simulink model "dyn_block"  (R2023b)
settings: Solver=VariableStepAuto  StartTime=0.0  StopTime=10.0  RelTol=1e-3
values from neighbouring files (symbols this model uses):
  i1 = sat.diaginertiamatrix(1, 1)    [set_params.m]
  i2 = sat.diaginertiamatrix(2, 2)    [set_params.m]
  i3 = sat.diaginertiamatrix(3, 3)    [set_params.m]
undefined symbols (not defined in the file or in its folder): compact, sat
libraries: aerolibutil x9, sharedtransform x2, shared6dof x1, sharedutil x1
settings Model: Creator=aryam  LastModifiedBy=aryam

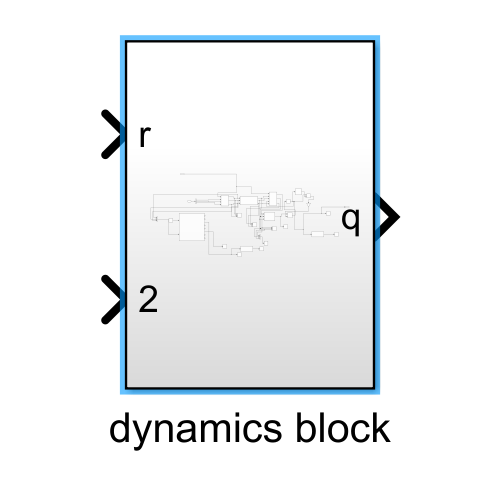
[thumbnail: Simulink's stored preview of the top-level diagram]
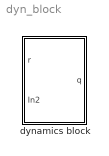
== system dyn_block ==
  dynamics block : Subsystem

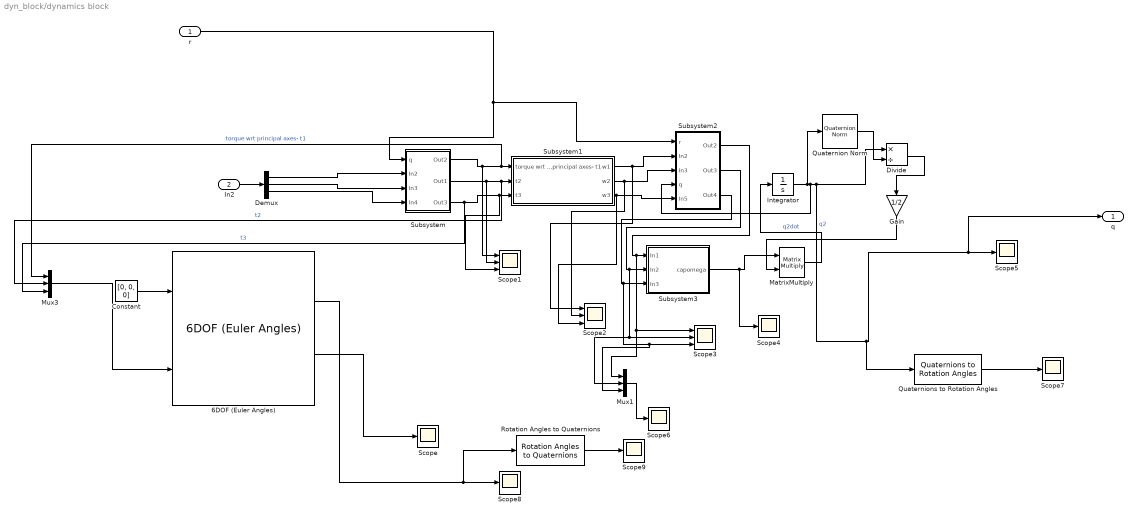
== system dyn_block/dynamics block ==
  r : Inport
  In2 : Inport  Port=2
  6DOF (Euler Angles) : shared6dof/6DOF (Euler Angles)  units=Metric (MKS)  mtype=Fixed  rep=Quaternion  xme_0=[0 0 0]  Vm_0=[0 0 0]  eul_0=[0 0 0]  pm_0=[0 0 0]  mass_0=1.0  mass_e=0.5  mass_f=2.0  inertia=sat.inertiamatrix  inertia_e=eye(3)  inertia_f=2*eye(3)  k_quat=1.0  vre_flag=on  abi_flag=off  aMode=0  xme_statename=''  Vm_statename=''  eul_statename=''  quat_statename=''  pm_statename=''  mass_statename=''
  Constant : Constant  Value=[0, 0, 0]
  Demux : Demux  Outputs=3
  Divide : Product  Inputs=*/
  Gain : Gain  Gain=1/2
  Integrator : Integrator  InitialCondition=compact(sat.initialorientation)
  MatrixMultiply : Product  Multiplication=Matrix(*)
  Mux1 : Mux  Inputs=3
  Mux3 : Mux  Inputs=3
  Quaternion Norm : sharedutil/Quaternion Norm  aMode=aMode
      settings: LibrarySourceBlock=|
      | aerolibutil/Quaternion
      | Norm
  Quaternions to Rotation Angles : sharedtransform/Quaternions to Rotation Angles  rotationOrder=ZYX  aMode=aMode
  Rotation Angles to Quaternions : sharedtransform/Rotation Angles to Quaternions  rotationOrder=ZYX  aMode=aMode
  Scope{,4..9} (7 alike) : Scope
  Scope1 : Scope  NumInputPorts=3
  Scope2 : Scope  NumInputPorts=3
  Scope3 : Scope  NumInputPorts=3
  Subsystem : Subsystem
  Subsystem1 : Subsystem
  Subsystem2 : Subsystem
  Subsystem3 : Subsystem
  q : Outport
  wires:
  Subsystem2/2(Out3) -> Scope3/2, Mux1/2, Subsystem3/2(In2)
  Subsystem2/3(Out4) -> Mux1/3, Scope3/3, Subsystem3/3(In3)
  Gain/1 -> MatrixMultiply/2
  Subsystem/1(Out2) -> Mux3/1, Subsystem1/1(torque wrt principal axes- t1), Scope1/1  "torque wrt principal axes- t1"
  Subsystem1/1(w1) -> Scope2/1, Subsystem2/2(In2)
  Subsystem3/1(capomega) -> Scope4/1, MatrixMultiply/1
  MatrixMultiply/1 -> Integrator/1  "q2dot"
  Subsystem/3(Out3) -> Mux3/3, Scope1/3, Subsystem1/3(t3)  "t3"
  r/1 -> Subsystem2/1(r), Subsystem/1(q)
  Subsystem1/2(w2) -> Scope2/2, Subsystem2/3(In3)
  Subsystem1/3(w3) -> Subsystem2/5(In5), Scope2/3
  Quaternion Norm/1 -> Divide/2
  Subsystem/2(Out1) -> Mux3/2, Subsystem1/2(t2), Scope1/2  "t2"
  Divide/1 -> Gain/1
  Integrator/1 -> Quaternions to Rotation Angles/1, q/1, Scope5/1, Divide/1, Subsystem2/4(q), Quaternion Norm/1  "q2"
  Subsystem2/1(Out2) -> Mux1/1, Scope3/1, Subsystem3/1(In1)
  Mux1/1 -> Scope6/1
  Mux3/1 -> 6DOF (Euler Angles)/2
  Constant/1 -> 6DOF (Euler Angles)/1
  6DOF (Euler Angles)/6 -> Scope/1
  Quaternions to Rotation Angles/1 -> Scope7/1
  6DOF (Euler Angles)/3 -> Rotation Angles to Quaternions/1, Scope8/1
  In2/1 -> Demux/1
  Demux/1 -> Subsystem/2(In2)
  Demux/2 -> Subsystem/3(In3)
  Demux/3 -> Subsystem/4(In4)
  Rotation Angles to Quaternions/1 -> Scope9/1

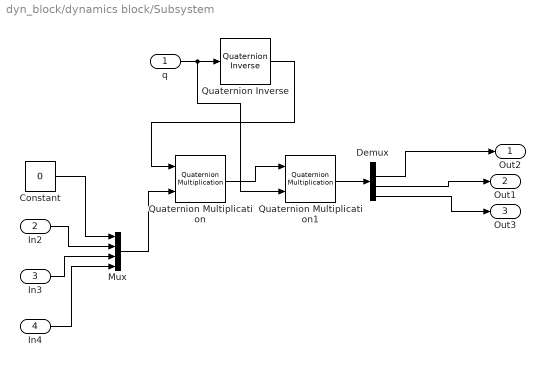
== system dyn_block/dynamics block/Subsystem ==
  q : Inport
  In2 : Inport  Port=2
  In3 : Inport  Port=3
  In4 : Inport  Port=4
  Constant : Constant  Value=0
  Demux : Demux
  Mux : Mux
  Quaternion Inverse : aerolibutil/Quaternion Inverse
  Quaternion Multiplication : aerolibutil/Quaternion Multiplication
  Quaternion Multiplication1 : aerolibutil/Quaternion Multiplication
  Out2 : Outport
  Out1 : Outport  Port=2
  Out3 : Outport  Port=3
  wires:
  Quaternion Multiplication/1 -> Quaternion Multiplication1/1
  Constant/1 -> Mux/1
  Mux/1 -> Quaternion Multiplication/2
  Demux/4 -> Out3/1
  q/1 -> Quaternion Multiplication1/2, Quaternion Inverse/1
  Quaternion Multiplication1/1 -> Demux/1
  Demux/3 -> Out1/1
  Demux/2 -> Out2/1
  Quaternion Inverse/1 -> Quaternion Multiplication/1
  In2/1 -> Mux/2
  In3/1 -> Mux/3
  In4/1 -> Mux/4

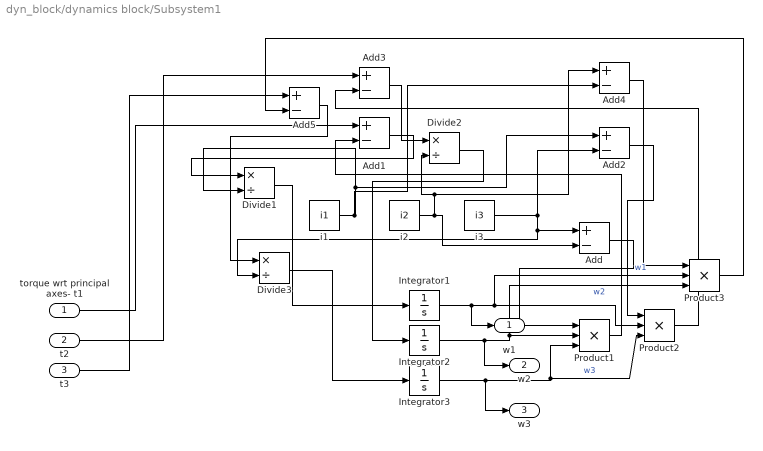
== system dyn_block/dynamics block/Subsystem1 ==
  torque wrt principal axes- t1 : Inport
  t2 : Inport  Port=2
  t3 : Inport  Port=3
  Add{,1..5} (6 alike) : Sum  Inputs=+-
  Divide1 : Product  Inputs=*/
  Divide2 : Product  Inputs=*/
  Divide3 : Product  Inputs=*/
  Integrator1 : Integrator  InitialCondition=sat.omegaprinc1
  Integrator2 : Integrator  InitialCondition=sat.omegaprinc2
  Integrator3 : Integrator  InitialCondition=sat.omegaprinc3
  Product1 : Product  Inputs=3
  Product2 : Product  Inputs=3
  Product3 : Product  Inputs=3
  i1 : Constant  Value=i1
  i2 : Constant  Value=i2
  i3 : Constant  Value=i3
  w1 : Outport
  w2 : Outport  Port=2
  w3 : Outport  Port=3
  wires:
  Integrator3/1 -> w3/1, Product2/3, Product1/3  "w3"
  Add3/1 -> Divide2/1
  Divide3/1 -> Integrator3/1
  Integrator1/1 -> w1/1, Product3/2, Product2/2  "w1"
  torque wrt principal axes- t1/1 -> Add1/1
  i1/1 -> Add4/2, Add2/1, Divide1/2
  Product3/1 -> Add5/2
  i2/1 -> Add4/1, Divide2/2, Add/2
  Integrator2/1 -> w2/1, Product3/3, Product1/2  "w2"
  Add1/1 -> Divide1/1
  Add5/1 -> Divide3/1
  Divide1/1 -> Integrator1/1
  Add2/1 -> Product2/1
  Add/1 -> Product1/1
  i3/1 -> Divide3/2, Add/1, Add2/2
  Product2/1 -> Add3/2
  Add4/1 -> Product3/1
  Divide2/1 -> Integrator2/1
  Product1/1 -> Add1/2
  t2/1 -> Add3/1
  t3/1 -> Add5/1

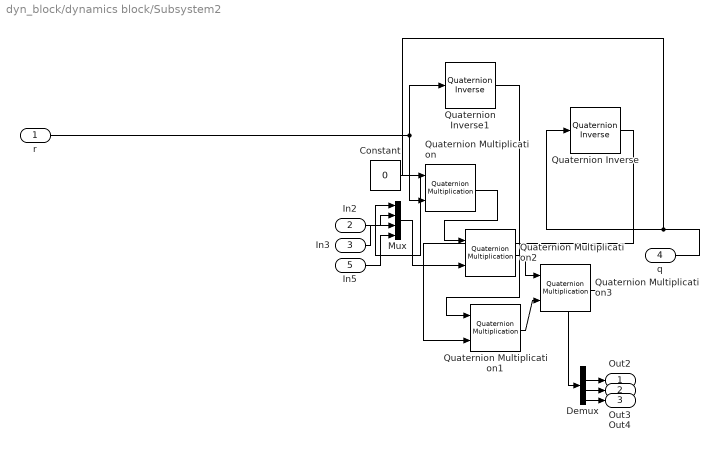
== system dyn_block/dynamics block/Subsystem2 ==
  r : Inport
  In2 : Inport  Port=2
  In3 : Inport  Port=3
  q : Inport  Port=4
  In5 : Inport  Port=5
  Constant : Constant  Value=0
  Demux : Demux
  Mux : Mux
  Quaternion Inverse : aerolibutil/Quaternion Inverse
  Quaternion Inverse1 : aerolibutil/Quaternion Inverse
  Quaternion Multiplication{,1..3} (4 alike) : aerolibutil/Quaternion Multiplication
  Out2 : Outport
  Out3 : Outport  Port=2
  Out4 : Outport  Port=3
  wires:
  Quaternion Multiplication2/1 -> Quaternion Multiplication3/1
  Constant/1 -> Mux/1
  Mux/1 -> Quaternion Multiplication2/2
  Quaternion Multiplication1/1 -> Quaternion Multiplication3/2
  Quaternion Inverse1/1 -> Quaternion Multiplication1/1
  Quaternion Multiplication3/1 -> Demux/1
  r/1 -> Quaternion Inverse1/1, Quaternion Multiplication/2
  Quaternion Multiplication/1 -> Quaternion Multiplication2/1
  q/1 -> Quaternion Multiplication/1, Quaternion Inverse/1
  Quaternion Inverse/1 -> Quaternion Multiplication1/2
  In5/1 -> Mux/4
  Demux/4 -> Out4/1
  Demux/2 -> Out2/1
  Demux/3 -> Out3/1
  In2/1 -> Mux/2
  In3/1 -> Mux/3

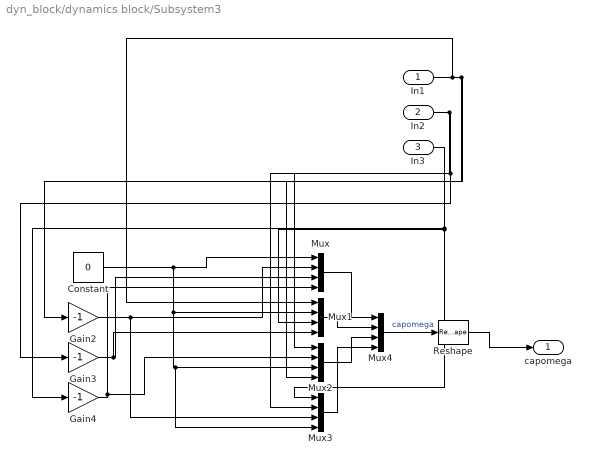
== system dyn_block/dynamics block/Subsystem3 ==
  In1 : Inport
  In2 : Inport  Port=2
  In3 : Inport  Port=3
  Constant : Constant  Value=0
  Gain2 : Gain  Gain=-1
  Gain3 : Gain  Gain=-1
  Gain4 : Gain  Gain=-1
  Mux{,1..4} (5 alike) : Mux
  Reshape : Reshape  OutputDimensionality=Customize  OutputDimensions=[4,4]
  capomega : Outport
  wires:
  Gain2/1 -> Mux3/3, Mux/2
  In1/1 -> Mux1/1, Mux2/4, Gain2/1
  Mux2/1 -> Mux4/3
  Constant/1 -> Mux3/4, Mux2/3, Mux1/2, Mux/1
  Mux3/1 -> Mux4/4
  Gain4/1 -> Mux2/2, Mux/4
  Gain3/1 -> Mux1/4, Mux/3
  In2/1 -> Mux3/2, Mux2/1, Gain3/1
  In3/1 -> Mux3/1, Mux1/3, Gain4/1
  Mux1/1 -> Mux4/2
  Mux/1 -> Mux4/1
  Mux4/1 -> Reshape/1  "capomega"
  Reshape/1 -> capomega/1
